simulink model "TLBO_2023"  (R2023b)
settings: Solver=ode45  StartTime=0.0  StopTime=6  MaxStep=1e-4  RelTol=1e-3  EnableMultiTasking=on
PreLoadFcn:
  | Ts_Power=1e-6;
  | Ts_Control=100e-6;
InitFcn:
  | Ts_Power=1e-6;
  | Ts_Control=100e-6;
  | Rtrans=0.142;
  | Xtrans=0.12e-6;
undefined symbols (not defined in the file): DiscIntNeverNeededParam, Ion, Lithium, sigbuilder_block
libraries: dspfdesign x80, spsSeriesRLCBranchLib x52, spsCurrentMeasurementLib x20, spsMeanLib x20, spsIdealSwitchLib x16, spsVoltageMeasurementLib x16, slpidlib x15, spsMosfetLib x14, dspindex x12, spsPWMGeneratorDCDCLib x10, spsGroundLib x10, spsBatteryLib x4
(part 3 of 4)

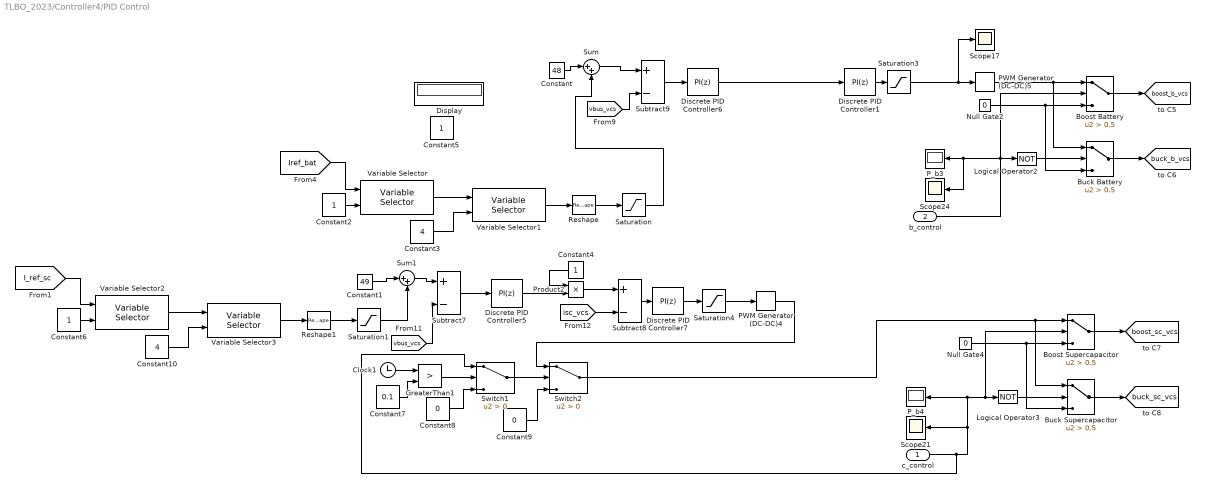
== system TLBO_2023/Controller4/PID Control ==
  c_control : Inport
  b_control : Inport  Port=2
  Boost Battery : Switch  Criteria=u2 > Threshold  Threshold=0.5  SaturateOnIntegerOverflow=off  InputSameDT=off
  Boost Supercapacitor : Switch  Criteria=u2 > Threshold  Threshold=0.5  SaturateOnIntegerOverflow=off  InputSameDT=off
  Buck Battery : Switch  Criteria=u2 > Threshold  Threshold=0.5  SaturateOnIntegerOverflow=off  InputSameDT=off
  Buck Supercapacitor : Switch  Criteria=u2 > Threshold  Threshold=0.5  SaturateOnIntegerOverflow=off  InputSameDT=off
  Clock1 : Clock
  Constant : Constant  Value=48
  Constant1 : Constant  Value=49
  Constant10 : Constant  Value=4
  Constant{2,4..6} (4 alike) : Constant
  Constant3 : Constant  Value=4
  Constant7 : Constant  Value=0.1
  Constant8 : Constant  Value=0
  Constant9 : Constant  Value=0
  Discrete PID Controller1 : slpidlib/PID Controller  Controller=PI  Form=Parallel  TimeDomain=Discrete-time  UseExternalTs=off  SampleTime=-1  IntegratorMethod=Forward Euler  FilterMethod=Forward Euler  ControllerParametersSource=internal  P=0.2  I=4  UseKiTs=off  D=1  N=100  UseFilter=on  TunerSelectOption=Transfer Function Based (PID Tuner App)  InitialConditionSource=internal  InitialConditionForIntegrator=0  InitialConditionForFilter=0  DifferentiatorICPrevScaledInput=0  ExternalReset=none  TrackingMode=off  Kt=1  LimitOutput=off  SatLimitsSource=internal  UpperSaturationLimit=inf  LowerSaturationLimit=-inf  LinearizeAsGain=off  AntiWindupMode=none  Kb=1  LimitIntegrator=off  UpperIntegratorSaturationLimit=inf  LowerIntegratorSaturationLimit=-inf  POutMin=[]  POutMax=[]  IOutMin=[]  IOutMax=[]  DOutMin=[]  DOutMax=[]  NOutMin=[]  NOutMax=[]  SumOutMin=[]  SumOutMax=[]  SaturationOutMin=[]  SaturationOutMax=[]  PParamMin=[]  PParamMax=[]  IParamMin=[]  IParamMax=[]  DParamMin=[]  DParamMax=[]  NParamMin=[]  NParamMax=[]  KbParamMin=[]  KbParamMax=[]  KtParamMin=[]  KtParamMax=[]  KbOutMin=[]  KbOutMax=[]  KtOutMin=[]  KtOutMax=[]  IntegratorOutMin=[]  IntegratorOutMax=[]  FilterOutMin=[]  FilterOutMax=[]  SumI1OutMin=[]  SumI1OutMax=[]  SumI2OutMin=[]  SumI2OutMax=[]  SumI3OutMin=[]  SumI3OutMax=[]  SumI4OutMin=[]  SumI4OutMax=[]  SumDOutMin=[]  SumDOutMax=[]  DifferentiatorOutMin=[]  DifferentiatorOutMax=[]  FilterDiffOutCoefMin=[]  FilterDiffOutCoefMax=[]  ReciprocalOutMin=[]  ReciprocalOutMax=[]  SumDenOutMin=[]  SumDenOutMax=[]  SumNumOutMin=[]  SumNumOutMax=[]  DivideOutMin=[]  DivideOutMax=[]  UdiffTsProdOutMin=[]  UdiffTsProdOutMax=[]  NTsProdOutMin=[]  NTsProdOutMax=[]  UintegralTsProdOutMin=[]  UintegralTsProdOutMax=[]  UngainTsProdOutMin=[]  UngainTsProdOutMax=[]  ClampingZeroOutDataTypeStr=Inherit: Inherit via back propagation  ClampingZeroOutMin=[]  ClampingZeroOutMax=[]  FilterDenConstantOutDataTypeStr=Inherit: Inherit via back propagation  FilterDenConstantOutMin=[]  FilterDenConstantOutMax=[]  PCopyOutDataTypeStr=Inherit: Inherit via back propagation  PCopyOutMin=[]  PCopyOutMax=[]  NCopyOutDataTypeStr=Inherit: Inherit via back propagation  NCopyOutMin=[]  NCopyOutMax=[]  IntegratorContinuousStateAttributes=''  IntegratorStateMustResolveToSignalObject=off  IntegratorRTWStateStorageClass=Auto  FilterContinuousStateAttributes=''  FilterStateMustResolveToSignalObject=off  FilterRTWStateStorageClass=Auto  ParallelPVariant=InternalParameters  IdealPVariant=Disabled  IVariant=InternalParameters  DVariant=Disabled  IntegratorVariant=Discrete  SatVariant=Disabled  AWVariant=Passthrough  PCopyVariant=Disabled  TRVariant=Disabled  FdbkBlocksVariant=Forward  IdealPFdbkVariant=Disabled  SatFdbkVariant=Disabled  DerivativeFilterVariant=Disabled  NVariant=Disabled  NCopyVariant=Disabled_SignalSpec  FilterICVariant=Disabled  IntegratorICVariant=InternalICs  ExternalResetVariant=Disabled  TRSumVariant=Passthrough  SumFdbkVariant=Disabled  SumVariant=Sum_PI  TsampFilterVariant=InternalTs  TsampNgainVariant=Passthrough  TsampIntegralVariant=Disabled_SignalSpec  ExternalSaturationOutDataTypeStr=Inherit: Same as second input
  Discrete PID Controller5 : slpidlib/PID Controller  Controller=PI  Form=Parallel  TimeDomain=Discrete-time  UseExternalTs=off  SampleTime=-1  IntegratorMethod=Forward Euler  FilterMethod=Forward Euler  ControllerParametersSource=internal  P=0  I=4  UseKiTs=off  D=1  N=100  UseFilter=on  TunerSelectOption=Transfer Function Based (PID Tuner App)  InitialConditionSource=internal  InitialConditionForIntegrator=0  InitialConditionForFilter=0  DifferentiatorICPrevScaledInput=0  ExternalReset=none  TrackingMode=off  Kt=1  LimitOutput=off  SatLimitsSource=internal  UpperSaturationLimit=inf  LowerSaturationLimit=-inf  LinearizeAsGain=off  AntiWindupMode=none  Kb=1  LimitIntegrator=off  UpperIntegratorSaturationLimit=inf  LowerIntegratorSaturationLimit=-inf  POutMin=[]  POutMax=[]  IOutMin=[]  IOutMax=[]  DOutMin=[]  DOutMax=[]  NOutMin=[]  NOutMax=[]  SumOutMin=[]  SumOutMax=[]  SaturationOutMin=[]  SaturationOutMax=[]  PParamMin=[]  PParamMax=[]  IParamMin=[]  IParamMax=[]  DParamMin=[]  DParamMax=[]  NParamMin=[]  NParamMax=[]  KbParamMin=[]  KbParamMax=[]  KtParamMin=[]  KtParamMax=[]  KbOutMin=[]  KbOutMax=[]  KtOutMin=[]  KtOutMax=[]  IntegratorOutMin=[]  IntegratorOutMax=[]  FilterOutMin=[]  FilterOutMax=[]  SumI1OutMin=[]  SumI1OutMax=[]  SumI2OutMin=[]  SumI2OutMax=[]  SumI3OutMin=[]  SumI3OutMax=[]  SumI4OutMin=[]  SumI4OutMax=[]  SumDOutMin=[]  SumDOutMax=[]  DifferentiatorOutMin=[]  DifferentiatorOutMax=[]  FilterDiffOutCoefMin=[]  FilterDiffOutCoefMax=[]  ReciprocalOutMin=[]  ReciprocalOutMax=[]  SumDenOutMin=[]  SumDenOutMax=[]  SumNumOutMin=[]  SumNumOutMax=[]  DivideOutMin=[]  DivideOutMax=[]  UdiffTsProdOutMin=[]  UdiffTsProdOutMax=[]  NTsProdOutMin=[]  NTsProdOutMax=[]  UintegralTsProdOutMin=[]  UintegralTsProdOutMax=[]  UngainTsProdOutMin=[]  UngainTsProdOutMax=[]  ClampingZeroOutDataTypeStr=Inherit: Inherit via back propagation  ClampingZeroOutMin=[]  ClampingZeroOutMax=[]  FilterDenConstantOutDataTypeStr=Inherit: Inherit via back propagation  FilterDenConstantOutMin=[]  FilterDenConstantOutMax=[]  PCopyOutDataTypeStr=Inherit: Inherit via back propagation  PCopyOutMin=[]  PCopyOutMax=[]  NCopyOutDataTypeStr=Inherit: Inherit via back propagation  NCopyOutMin=[]  NCopyOutMax=[]  IntegratorContinuousStateAttributes=''  IntegratorStateMustResolveToSignalObject=off  IntegratorRTWStateStorageClass=Auto  FilterContinuousStateAttributes=''  FilterStateMustResolveToSignalObject=off  FilterRTWStateStorageClass=Auto  ParallelPVariant=InternalParameters  IdealPVariant=Disabled  IVariant=InternalParameters  DVariant=Disabled  IntegratorVariant=Discrete  SatVariant=Disabled  AWVariant=Passthrough  PCopyVariant=Disabled  TRVariant=Disabled  FdbkBlocksVariant=Forward  IdealPFdbkVariant=Disabled  SatFdbkVariant=Disabled  DerivativeFilterVariant=Disabled  NVariant=Disabled  NCopyVariant=Disabled_SignalSpec  FilterICVariant=Disabled  IntegratorICVariant=InternalICs  ExternalResetVariant=Disabled  TRSumVariant=Passthrough  SumFdbkVariant=Disabled  SumVariant=Sum_PI  TsampFilterVariant=InternalTs  TsampNgainVariant=Passthrough  TsampIntegralVariant=Disabled_SignalSpec  ExternalSaturationOutDataTypeStr=Inherit: Same as second input
  Discrete PID Controller6 : slpidlib/PID Controller  Controller=PI  Form=Parallel  TimeDomain=Discrete-time  UseExternalTs=off  SampleTime=-1  IntegratorMethod=Forward Euler  FilterMethod=Forward Euler  ControllerParametersSource=internal  P=0  I=1  UseKiTs=off  D=1  N=100  UseFilter=on  TunerSelectOption=Transfer Function Based (PID Tuner App)  InitialConditionSource=internal  InitialConditionForIntegrator=0  InitialConditionForFilter=0  DifferentiatorICPrevScaledInput=0  ExternalReset=none  TrackingMode=off  Kt=1  LimitOutput=off  SatLimitsSource=internal  UpperSaturationLimit=inf  LowerSaturationLimit=-inf  LinearizeAsGain=off  AntiWindupMode=none  Kb=1  LimitIntegrator=off  UpperIntegratorSaturationLimit=inf  LowerIntegratorSaturationLimit=-inf  POutMin=[]  POutMax=[]  IOutMin=[]  IOutMax=[]  DOutMin=[]  DOutMax=[]  NOutMin=[]  NOutMax=[]  SumOutMin=[]  SumOutMax=[]  SaturationOutMin=[]  SaturationOutMax=[]  PParamMin=[]  PParamMax=[]  IParamMin=[]  IParamMax=[]  DParamMin=[]  DParamMax=[]  NParamMin=[]  NParamMax=[]  KbParamMin=[]  KbParamMax=[]  KtParamMin=[]  KtParamMax=[]  KbOutMin=[]  KbOutMax=[]  KtOutMin=[]  KtOutMax=[]  IntegratorOutMin=[]  IntegratorOutMax=[]  FilterOutMin=[]  FilterOutMax=[]  SumI1OutMin=[]  SumI1OutMax=[]  SumI2OutMin=[]  SumI2OutMax=[]  SumI3OutMin=[]  SumI3OutMax=[]  SumI4OutMin=[]  SumI4OutMax=[]  SumDOutMin=[]  SumDOutMax=[]  DifferentiatorOutMin=[]  DifferentiatorOutMax=[]  FilterDiffOutCoefMin=[]  FilterDiffOutCoefMax=[]  ReciprocalOutMin=[]  ReciprocalOutMax=[]  SumDenOutMin=[]  SumDenOutMax=[]  SumNumOutMin=[]  SumNumOutMax=[]  DivideOutMin=[]  DivideOutMax=[]  UdiffTsProdOutMin=[]  UdiffTsProdOutMax=[]  NTsProdOutMin=[]  NTsProdOutMax=[]  UintegralTsProdOutMin=[]  UintegralTsProdOutMax=[]  UngainTsProdOutMin=[]  UngainTsProdOutMax=[]  ClampingZeroOutDataTypeStr=Inherit: Inherit via back propagation  ClampingZeroOutMin=[]  ClampingZeroOutMax=[]  FilterDenConstantOutDataTypeStr=Inherit: Inherit via back propagation  FilterDenConstantOutMin=[]  FilterDenConstantOutMax=[]  PCopyOutDataTypeStr=Inherit: Inherit via back propagation  PCopyOutMin=[]  PCopyOutMax=[]  NCopyOutDataTypeStr=Inherit: Inherit via back propagation  NCopyOutMin=[]  NCopyOutMax=[]  IntegratorContinuousStateAttributes=''  IntegratorStateMustResolveToSignalObject=off  IntegratorRTWStateStorageClass=Auto  FilterContinuousStateAttributes=''  FilterStateMustResolveToSignalObject=off  FilterRTWStateStorageClass=Auto  ParallelPVariant=InternalParameters  IdealPVariant=Disabled  IVariant=InternalParameters  DVariant=Disabled  IntegratorVariant=Discrete  SatVariant=Disabled  AWVariant=Passthrough  PCopyVariant=Disabled  TRVariant=Disabled  FdbkBlocksVariant=Forward  IdealPFdbkVariant=Disabled  SatFdbkVariant=Disabled  DerivativeFilterVariant=Disabled  NVariant=Disabled  NCopyVariant=Disabled_SignalSpec  FilterICVariant=Disabled  IntegratorICVariant=InternalICs  ExternalResetVariant=Disabled  TRSumVariant=Passthrough  SumFdbkVariant=Disabled  SumVariant=Sum_PI  TsampFilterVariant=InternalTs  TsampNgainVariant=Passthrough  TsampIntegralVariant=Disabled_SignalSpec  ExternalSaturationOutDataTypeStr=Inherit: Same as second input
  Discrete PID Controller7 : slpidlib/PID Controller  Controller=PI  Form=Parallel  TimeDomain=Discrete-time  UseExternalTs=off  SampleTime=-1  IntegratorMethod=Forward Euler  FilterMethod=Forward Euler  ControllerParametersSource=internal  P=0.2  I=4  UseKiTs=off  D=1  N=100  UseFilter=on  TunerSelectOption=Transfer Function Based (PID Tuner App)  InitialConditionSource=internal  InitialConditionForIntegrator=0  InitialConditionForFilter=0  DifferentiatorICPrevScaledInput=0  ExternalReset=none  TrackingMode=off  Kt=1  LimitOutput=off  SatLimitsSource=internal  UpperSaturationLimit=inf  LowerSaturationLimit=-inf  LinearizeAsGain=off  AntiWindupMode=none  Kb=1  LimitIntegrator=off  UpperIntegratorSaturationLimit=inf  LowerIntegratorSaturationLimit=-inf  POutMin=[]  POutMax=[]  IOutMin=[]  IOutMax=[]  DOutMin=[]  DOutMax=[]  NOutMin=[]  NOutMax=[]  SumOutMin=[]  SumOutMax=[]  SaturationOutMin=[]  SaturationOutMax=[]  PParamMin=[]  PParamMax=[]  IParamMin=[]  IParamMax=[]  DParamMin=[]  DParamMax=[]  NParamMin=[]  NParamMax=[]  KbParamMin=[]  KbParamMax=[]  KtParamMin=[]  KtParamMax=[]  KbOutMin=[]  KbOutMax=[]  KtOutMin=[]  KtOutMax=[]  IntegratorOutMin=[]  IntegratorOutMax=[]  FilterOutMin=[]  FilterOutMax=[]  SumI1OutMin=[]  SumI1OutMax=[]  SumI2OutMin=[]  SumI2OutMax=[]  SumI3OutMin=[]  SumI3OutMax=[]  SumI4OutMin=[]  SumI4OutMax=[]  SumDOutMin=[]  SumDOutMax=[]  DifferentiatorOutMin=[]  DifferentiatorOutMax=[]  FilterDiffOutCoefMin=[]  FilterDiffOutCoefMax=[]  ReciprocalOutMin=[]  ReciprocalOutMax=[]  SumDenOutMin=[]  SumDenOutMax=[]  SumNumOutMin=[]  SumNumOutMax=[]  DivideOutMin=[]  DivideOutMax=[]  UdiffTsProdOutMin=[]  UdiffTsProdOutMax=[]  NTsProdOutMin=[]  NTsProdOutMax=[]  UintegralTsProdOutMin=[]  UintegralTsProdOutMax=[]  UngainTsProdOutMin=[]  UngainTsProdOutMax=[]  ClampingZeroOutDataTypeStr=Inherit: Inherit via back propagation  ClampingZeroOutMin=[]  ClampingZeroOutMax=[]  FilterDenConstantOutDataTypeStr=Inherit: Inherit via back propagation  FilterDenConstantOutMin=[]  FilterDenConstantOutMax=[]  PCopyOutDataTypeStr=Inherit: Inherit via back propagation  PCopyOutMin=[]  PCopyOutMax=[]  NCopyOutDataTypeStr=Inherit: Inherit via back propagation  NCopyOutMin=[]  NCopyOutMax=[]  IntegratorContinuousStateAttributes=''  IntegratorStateMustResolveToSignalObject=off  IntegratorRTWStateStorageClass=Auto  FilterContinuousStateAttributes=''  FilterStateMustResolveToSignalObject=off  FilterRTWStateStorageClass=Auto  ParallelPVariant=InternalParameters  IdealPVariant=Disabled  IVariant=InternalParameters  DVariant=Disabled  IntegratorVariant=Discrete  SatVariant=Disabled  AWVariant=Passthrough  PCopyVariant=Disabled  TRVariant=Disabled  FdbkBlocksVariant=Forward  IdealPFdbkVariant=Disabled  SatFdbkVariant=Disabled  DerivativeFilterVariant=Disabled  NVariant=Disabled  NCopyVariant=Disabled_SignalSpec  FilterICVariant=Disabled  IntegratorICVariant=InternalICs  ExternalResetVariant=Disabled  TRSumVariant=Passthrough  SumFdbkVariant=Disabled  SumVariant=Sum_PI  TsampFilterVariant=InternalTs  TsampNgainVariant=Passthrough  TsampIntegralVariant=Disabled_SignalSpec  ExternalSaturationOutDataTypeStr=Inherit: Same as second input
  Display : Display
  GreaterThan1 : RelationalOperator  Operator=>  OutDataTypeStr=boolean  RndMeth=Simplest  InputSameDT=off
  Logical Operator2 : Logic  Operator=NOT  AllPortsSameDT=off  OutDataTypeStr=boolean
  Logical Operator3 : Logic  Operator=NOT  AllPortsSameDT=off  OutDataTypeStr=boolean
  Null Gate2 : Constant  Value=0
  Null Gate4 : Constant  Value=0
  PWM Generator (DC-DC)4 : spsPWMGeneratorDCDCLib/PWM Generator (DC-DC)  Fsw=10e3  Ts=0
  PWM Generator (DC-DC)5 : spsPWMGeneratorDCDCLib/PWM Generator (DC-DC)  Fsw=10e3  Ts=0
  P_b3 : Display
      settings: Format=binary (Stored Integer)  Decimation=1000
  P_b4 : Display
      settings: Format=binary (Stored Integer)  Decimation=1000
  Product2 : Product
  Reshape : Reshape
  Reshape1 : Reshape
  Saturation : Saturate
  Saturation1 : Saturate
  Saturation3 : Saturate  UpperLimit=0.8  LowerLimit=0  ZeroCross=off
  Saturation4 : Saturate  UpperLimit=0.8  LowerLimit=0  ZeroCross=off
  Scope17 : Scope
  Scope21 : Scope
  Scope24 : Scope
  Subtract7 : Sum  Inputs=+-
  Subtract8 : Sum  Inputs=+-
  Subtract9 : Sum  Inputs=+-
  Sum : Sum  Inputs=|++
  Sum1 : Sum  Inputs=|++
  Switch1 : Switch  Criteria=u2 > Threshold  SaturateOnIntegerOverflow=off  InputSameDT=off
  Switch2 : Switch  Criteria=u2 > Threshold  SaturateOnIntegerOverflow=off  InputSameDT=off
  Variable Selector : dspindex/Variable Selector  NumInputs=1  rowsOrCols=Rows  IdxMode=Variable  Elements=[1 3]  ZerOneIdxMode=One-based  errmode=Clip Index  FillMode=on  FillValues=0
  Variable Selector1 : dspindex/Variable Selector  NumInputs=1  rowsOrCols=Columns  IdxMode=Variable  Elements=[1 3]  ZerOneIdxMode=One-based  errmode=Clip Index  FillMode=on  FillValues=0
  Variable Selector2 : dspindex/Variable Selector  NumInputs=1  rowsOrCols=Rows  IdxMode=Variable  Elements=[1 3]  ZerOneIdxMode=One-based  errmode=Clip Index  FillMode=on  FillValues=0
  Variable Selector3 : dspindex/Variable Selector  NumInputs=1  rowsOrCols=Columns  IdxMode=Variable  Elements=[1 3]  ZerOneIdxMode=One-based  errmode=Clip Index  FillMode=on  FillValues=0
  tag scope: boost_b_vcs=global, boost_sc_vcs=global, buck_b_vcs=global, buck_sc_vcs=global
  wires:
  Buck Battery/1 -> [buck_b_vcs]
  Null Gate2/1 -> Boost Battery/3, Buck Battery/3
  b_control/1 -> Scope24/1, P_b3/1, Logical Operator2/1, Boost Battery/2
  Boost Battery/1 -> [boost_b_vcs]
  PWM Generator (DC-DC)5/1 -> Buck Battery/1, Boost Battery/1
  Logical Operator2/1 -> Buck Battery/2
  [vbus_vcs] -> Subtract9/2
  Buck Supercapacitor/1 -> [buck_sc_vcs]
  Null Gate4/1 -> Buck Supercapacitor/3, Boost Supercapacitor/3
  Boost Supercapacitor/1 -> [boost_sc_vcs]
  Subtract7/1 -> Discrete PID Controller5/1
  [vbus_vcs] -> Subtract7/2
  Saturation4/1 -> PWM Generator (DC-DC)4/1
  Saturation3/1 -> Scope17/1, PWM Generator (DC-DC)5/1
  [isc_vcs] -> Subtract8/2
  Product2/1 -> Subtract8/1
  Discrete PID Controller5/1 -> Product2/2
  Constant4/1 -> Product2/1
  Subtract8/1 -> Discrete PID Controller7/1
  Discrete PID Controller7/1 -> Saturation4/1
  Subtract9/1 -> Discrete PID Controller6/1
  Discrete PID Controller1/1 -> Saturation3/1
  Reshape/1 -> Saturation/1
  Variable Selector/1 -> Variable Selector1/1
  Constant3/1 -> Variable Selector1/2
  [Iref_bat] -> Variable Selector/1
  Variable Selector1/1 -> Reshape/1
  Constant2/1 -> Variable Selector/2
  Discrete PID Controller6/1 -> Discrete PID Controller1/1
  Constant/1 -> Sum/1
  Sum/1 -> Subtract9/1
  c_control/1 -> Switch1/1, Scope21/1, P_b4/1, Boost Supercapacitor/2, Logical Operator3/1
  Logical Operator3/1 -> Buck Supercapacitor/2
  PWM Generator (DC-DC)4/1 -> Switch2/1
  GreaterThan1/1 -> Switch1/2
  Clock1/1 -> GreaterThan1/1
  Constant9/1 -> Switch2/3
  Constant8/1 -> Switch1/3
  Constant7/1 -> GreaterThan1/2
  Switch1/1 -> Switch2/2
  Switch2/1 -> Buck Supercapacitor/1, Boost Supercapacitor/1
  Saturation/1 -> Sum/2
  Variable Selector3/1 -> Reshape1/1
  Reshape1/1 -> Saturation1/1
  Variable Selector2/1 -> Variable Selector3/1
  Constant10/1 -> Variable Selector3/2
  Constant6/1 -> Variable Selector2/2
  [I_ref_sc] -> Variable Selector2/1
  Constant1/1 -> Sum1/1
  Saturation1/1 -> Sum1/2
  Sum1/1 -> Subtract7/1

== system TLBO_2023/DC Load 1_2/Load Control ==
  Demux : Demux  Tag=STV Demux  Outputs=5
      settings: DisplayOption=none
  FromWs : FromWorkspace  Tag=STV FromWs  VariableName=tuvar
      SigBuilderData=|
      | common.afterFinalStr = 'Extrapolate'
      | common.sampleTime = '0'
      | dataSet(1).timeRange = [0 6]
      | dataSet(1).name = 'Constant Irradiance'
      | dataSet(2).timeRange = [0 6]
      | dataSet(2).name = 'Step Irradiance'
      | dataSet(3).timeRange = [0 6]
      | dataSet(3).name = 'Load Switch Control'
      | sbobj.Groups(1).Name = 'Constant Irradiance'
      | sbobj.Groups(1).Signals(1).Name = 'S1'
      | sbobj.Groups(1).Signals(1).XData = [0 6]
      | sbobj.Groups(1).Signals(1).YData = [1000 1000]
      | sbobj.Groups(1).Signals(2).Name = 'S2'
      | sbobj.Groups(1).Signals(2).XData = [0 3 3 6]
      | sbobj.Groups(1).Signals(2).YData = [0 0 1 1]
      | sbobj.Groups(1).Signals(3).Name = 'S3'
      | sbobj.Groups(1).Signals(3).XData = [0 3 3 6]
      | sbobj.Groups(1).Signals(3).YData = [0 0 1 1]
      | sbobj.Groups(1).Signals(4).Name = 'S4'
      | sbobj.Groups(1).Signals(4).XData = [0 3 3 6]
      | sbobj.Groups(1).Signals(4).YData = [0 0 1 1]
      | sbobj.Groups(1).Signals(5).Name = 'Signal 1'
      | sbobj.Groups(1).Signals(5).XData = [0 6]
      | sbobj.Groups(1).Signals(5).YData = [0 0]
      | sbobj.Groups(1).TimeRange = [0 6]
      | sbobj.Groups(2).Name = 'Step Irradiance'
      | sbobj.Groups(2).Signals(1).Name = 'S1'
      | sbobj.Groups(2).Signals(1).XData = [0 0.252 0.252 6]
      | sbobj.Groups(2).Signals(1).YData = [600 600 1000 1000]
      | sbobj.Groups(2).Signals(2).Name = 'S2'
      | sbobj.Groups(2).Signals(2).XData = [0 3 3 6]
      | sbobj.Groups(2).Signals(2).YData = [0 0 1 1]
      | sbobj.Groups(2).Signals(3).Name = 'S3'
      | sbobj.Groups(2).Signals(3).XData = [0 3 3 6]
      | sbobj.Groups(2).Signals(3).YData = [0 0 1 1]
      | sbobj.Groups(2).Signals(4).Name = 'S4'
      | sbobj.Groups(2).Signals(4).XData = [0 3 3 6]
      | sbobj.Groups(2).Signals(4).YData = [0 0 1 1]
      | sbobj.Groups(2).Signals(5).Name = 'Signal 1'
      | sbobj.Groups(2).Signals(5).XData = [0 6]
      | sbobj.Groups(2).Signals(5).YData = [0 0]
      | sbobj.Groups(2).TimeRange = [0 6]
      | sbobj.Groups(3).Name = 'Load Switch Control'
      | sbobj.Groups(3).Signals(1).Name = 'S1'
      | sbobj.Groups(3).Signals(1).XData = [0 2.995 2.995 3.995 3.995 6]
      | sbobj.Groups(3).Signals(1).YData = [-0.01 -0.01 1 1 0 0]
      | sbobj.Groups(3).Signals(2).Name = 'S2'
      | sbobj.Groups(3).Signals(2).XData = [0 2 3 6]
      | sbobj.Groups(3).Signals(2).YData = [0 0 0 0]
      | sbobj.Groups(3).Signals(3).Name = 'S3'
      | sbobj.Groups(3).Signals(3).XData = [0 3 3 4 4 6]
      | sbobj.Groups(3).Signals(3).YData = [0 0 1 1 0 0]
      | sbobj.Groups(3).Signals(4).Name = 'S4'
      | sbobj.Groups(3).Signals(4).XData = [0 3 4 5 6]
      | sbobj.Groups(3).Signals(4).YData = [0 0 0 0 0]
      | sbobj.Groups(3).Signals(5).Name = 'Signal 1'
      | sbobj.Groups(3).Signals(5).XData = [0 6]
      | sbobj.Groups(3).Signals(5).YData = [0 0]
      | sbobj.Groups(3).TimeRange = [0 6]
  S1 : Outport  Tag=STV Outport  VectorParamsAs1DForOutWhenUnconnected=off
  S2 : Outport  Tag=STV Outport  Port=2  VectorParamsAs1DForOutWhenUnconnected=off
  S3 : Outport  Tag=STV Outport  Port=3  VectorParamsAs1DForOutWhenUnconnected=off
  S4 : Outport  Tag=STV Outport  Port=4  VectorParamsAs1DForOutWhenUnconnected=off
  Signal 1 : Outport  Tag=STV Outport  Port=5
  wires:
  Demux/1 -> S1/1
  FromWs/1 -> Demux/1
  Demux/2 -> S2/1
  Demux/3 -> S3/1
  Demux/4 -> S4/1
  Demux/5 -> Signal 1/1

== system TLBO_2023/DC Load 1_4/Load Control ==
  Demux : Demux  Tag=STV Demux  Outputs=5
      settings: DisplayOption=none
  FromWs : FromWorkspace  Tag=STV FromWs  VariableName=tuvar
      SigBuilderData=|
      | common.afterFinalStr = 'Extrapolate'
      | common.sampleTime = '0'
      | dataSet(1).timeRange = [0 6]
      | dataSet(1).name = 'Constant Irradiance'
      | dataSet(2).timeRange = [0 6]
      | dataSet(2).name = 'Step Irradiance'
      | dataSet(3).timeRange = [0 6]
      | dataSet(3).name = 'Load Switch Control'
      | sbobj.Groups(1).Name = 'Constant Irradiance'
      | sbobj.Groups(1).Signals(1).Name = 'S1'
      | sbobj.Groups(1).Signals(1).XData = [0 6]
      | sbobj.Groups(1).Signals(1).YData = [1000 1000]
      | sbobj.Groups(1).Signals(2).Name = 'S2'
      | sbobj.Groups(1).Signals(2).XData = [0 3 3 6]
      | sbobj.Groups(1).Signals(2).YData = [0 0 1 1]
      | sbobj.Groups(1).Signals(3).Name = 'S3'
      | sbobj.Groups(1).Signals(3).XData = [0 3 3 6]
      | sbobj.Groups(1).Signals(3).YData = [0 0 1 1]
      | sbobj.Groups(1).Signals(4).Name = 'S4'
      | sbobj.Groups(1).Signals(4).XData = [0 3 3 6]
      | sbobj.Groups(1).Signals(4).YData = [0 0 1 1]
      | sbobj.Groups(1).Signals(5).Name = 'Signal 1'
      | sbobj.Groups(1).Signals(5).XData = [0 6]
      | sbobj.Groups(1).Signals(5).YData = [0 0]
      | sbobj.Groups(1).TimeRange = [0 6]
      | sbobj.Groups(2).Name = 'Step Irradiance'
      | sbobj.Groups(2).Signals(1).Name = 'S1'
      | sbobj.Groups(2).Signals(1).XData = [0 0.252 0.252 6]
      | sbobj.Groups(2).Signals(1).YData = [600 600 1000 1000]
      | sbobj.Groups(2).Signals(2).Name = 'S2'
      | sbobj.Groups(2).Signals(2).XData = [0 3 3 6]
      | sbobj.Groups(2).Signals(2).YData = [0 0 1 1]
      | sbobj.Groups(2).Signals(3).Name = 'S3'
      | sbobj.Groups(2).Signals(3).XData = [0 3 3 6]
      | sbobj.Groups(2).Signals(3).YData = [0 0 1 1]
      | sbobj.Groups(2).Signals(4).Name = 'S4'
      | sbobj.Groups(2).Signals(4).XData = [0 3 3 6]
      | sbobj.Groups(2).Signals(4).YData = [0 0 1 1]
      | sbobj.Groups(2).Signals(5).Name = 'Signal 1'
      | sbobj.Groups(2).Signals(5).XData = [0 6]
      | sbobj.Groups(2).Signals(5).YData = [0 0]
      | sbobj.Groups(2).TimeRange = [0 6]
      | sbobj.Groups(3).Name = 'Load Switch Control'
      | sbobj.Groups(3).Signals(1).Name = 'S1'
      | sbobj.Groups(3).Signals(1).XData = [0 0.06 0.06 0.99 0.99 6]
      | sbobj.Groups(3).Signals(1).YData = [-0.01 -0.01 0.99 1.01 0 0]
      | sbobj.Groups(3).Signals(2).Name = 'S2'
      | sbobj.Groups(3).Signals(2).XData = [0 2 3 6]
      | sbobj.Groups(3).Signals(2).YData = [0 0 0 0]
      | sbobj.Groups(3).Signals(3).Name = 'S3'
      | sbobj.Groups(3).Signals(3).XData = [0 3 3 4 4 6]
      | sbobj.Groups(3).Signals(3).YData = [0 0 1 1 0 0]
      | sbobj.Groups(3).Signals(4).Name = 'S4'
      | sbobj.Groups(3).Signals(4).XData = [0 3 4 5 6]
      | sbobj.Groups(3).Signals(4).YData = [0 0 0 0 0]
      | sbobj.Groups(3).Signals(5).Name = 'Signal 1'
      | sbobj.Groups(3).Signals(5).XData = [0 6]
      | sbobj.Groups(3).Signals(5).YData = [0 0]
      | sbobj.Groups(3).TimeRange = [0 6]
  S1 : Outport  Tag=STV Outport  VectorParamsAs1DForOutWhenUnconnected=off
  S2 : Outport  Tag=STV Outport  Port=2  VectorParamsAs1DForOutWhenUnconnected=off
  S3 : Outport  Tag=STV Outport  Port=3  VectorParamsAs1DForOutWhenUnconnected=off
  S4 : Outport  Tag=STV Outport  Port=4  VectorParamsAs1DForOutWhenUnconnected=off
  Signal 1 : Outport  Tag=STV Outport  Port=5
  wires:
  Demux/1 -> S1/1
  FromWs/1 -> Demux/1
  Demux/2 -> S2/1
  Demux/3 -> S3/1
  Demux/4 -> S4/1
  Demux/5 -> Signal 1/1

== system TLBO_2023/DC Load 2_3/Load Control ==
  Demux : Demux  Tag=STV Demux  Outputs=5
      settings: DisplayOption=none
  FromWs : FromWorkspace  Tag=STV FromWs  VariableName=tuvar
      SigBuilderData=|
      | common.afterFinalStr = 'Extrapolate'
      | common.sampleTime = '0'
      | dataSet(1).timeRange = [0 6]
      | dataSet(1).name = 'Constant Irradiance'
      | dataSet(2).timeRange = [0 6]
      | dataSet(2).name = 'Step Irradiance'
      | dataSet(3).timeRange = [0 6]
      | dataSet(3).name = 'Load Switch Control'
      | sbobj.Groups(1).Name = 'Constant Irradiance'
      | sbobj.Groups(1).Signals(1).Name = 'S1'
      | sbobj.Groups(1).Signals(1).XData = [0 6]
      | sbobj.Groups(1).Signals(1).YData = [1000 1000]
      | sbobj.Groups(1).Signals(2).Name = 'S2'
      | sbobj.Groups(1).Signals(2).XData = [0 3 3 6]
      | sbobj.Groups(1).Signals(2).YData = [0 0 1 1]
      | sbobj.Groups(1).Signals(3).Name = 'S3'
      | sbobj.Groups(1).Signals(3).XData = [0 3 3 6]
      | sbobj.Groups(1).Signals(3).YData = [0 0 1 1]
      | sbobj.Groups(1).Signals(4).Name = 'S4'
      | sbobj.Groups(1).Signals(4).XData = [0 3 3 6]
      | sbobj.Groups(1).Signals(4).YData = [0 0 1 1]
      | sbobj.Groups(1).Signals(5).Name = 'Signal 1'
      | sbobj.Groups(1).Signals(5).XData = [0 6]
      | sbobj.Groups(1).Signals(5).YData = [0 0]
      | sbobj.Groups(1).TimeRange = [0 6]
      | sbobj.Groups(2).Name = 'Step Irradiance'
      | sbobj.Groups(2).Signals(1).Name = 'S1'
      | sbobj.Groups(2).Signals(1).XData = [0 0.252 0.252 6]
      | sbobj.Groups(2).Signals(1).YData = [600 600 1000 1000]
      | sbobj.Groups(2).Signals(2).Name = 'S2'
      | sbobj.Groups(2).Signals(2).XData = [0 3 3 6]
      | sbobj.Groups(2).Signals(2).YData = [0 0 1 1]
      | sbobj.Groups(2).Signals(3).Name = 'S3'
      | sbobj.Groups(2).Signals(3).XData = [0 3 3 6]
      | sbobj.Groups(2).Signals(3).YData = [0 0 1 1]
      | sbobj.Groups(2).Signals(4).Name = 'S4'
      | sbobj.Groups(2).Signals(4).XData = [0 3 3 6]
      | sbobj.Groups(2).Signals(4).YData = [0 0 1 1]
      | sbobj.Groups(2).Signals(5).Name = 'Signal 1'
      | sbobj.Groups(2).Signals(5).XData = [0 6]
      | sbobj.Groups(2).Signals(5).YData = [0 0]
      | sbobj.Groups(2).TimeRange = [0 6]
      | sbobj.Groups(3).Name = 'Load Switch Control'
      | sbobj.Groups(3).Signals(1).Name = 'S1'
      | sbobj.Groups(3).Signals(1).XData = [0 2.005 2.005 3.01 3.01 6]
      | sbobj.Groups(3).Signals(1).YData = [-0.01 -0.01 1 1.01 0 0]
      | sbobj.Groups(3).Signals(2).Name = 'S2'
      | sbobj.Groups(3).Signals(2).XData = [0 2 3 6]
      | sbobj.Groups(3).Signals(2).YData = [0 0 0 0]
      | sbobj.Groups(3).Signals(3).Name = 'S3'
      | sbobj.Groups(3).Signals(3).XData = [0 3 3 4 4 6]
      | sbobj.Groups(3).Signals(3).YData = [0 0 1 1 0 0]
      | sbobj.Groups(3).Signals(4).Name = 'S4'
      | sbobj.Groups(3).Signals(4).XData = [0 3 4 5 6]
      | sbobj.Groups(3).Signals(4).YData = [0 0 0 0 0]
      | sbobj.Groups(3).Signals(5).Name = 'Signal 1'
      | sbobj.Groups(3).Signals(5).XData = [0 6]
      | sbobj.Groups(3).Signals(5).YData = [0 0]
      | sbobj.Groups(3).TimeRange = [0 6]
  S1 : Outport  Tag=STV Outport  VectorParamsAs1DForOutWhenUnconnected=off
  S2 : Outport  Tag=STV Outport  Port=2  VectorParamsAs1DForOutWhenUnconnected=off
  S3 : Outport  Tag=STV Outport  Port=3  VectorParamsAs1DForOutWhenUnconnected=off
  S4 : Outport  Tag=STV Outport  Port=4  VectorParamsAs1DForOutWhenUnconnected=off
  Signal 1 : Outport  Tag=STV Outport  Port=5
  wires:
  Demux/1 -> S1/1
  FromWs/1 -> Demux/1
  Demux/2 -> S2/1
  Demux/3 -> S3/1
  Demux/4 -> S4/1
  Demux/5 -> Signal 1/1

== system TLBO_2023/DC Load 3_4/Load Control ==
  Demux : Demux  Tag=STV Demux  Outputs=5
      settings: DisplayOption=none
  FromWs : FromWorkspace  Tag=STV FromWs  VariableName=tuvar
      SigBuilderData=|
      | common.afterFinalStr = 'Extrapolate'
      | common.sampleTime = '0'
      | dataSet(1).timeRange = [0 6]
      | dataSet(1).name = 'Constant Irradiance'
      | dataSet(2).timeRange = [0 6]
      | dataSet(2).name = 'Step Irradiance'
      | dataSet(3).timeRange = [0 6]
      | dataSet(3).name = 'Load Switch Control'
      | sbobj.Groups(1).Name = 'Constant Irradiance'
      | sbobj.Groups(1).Signals(1).Name = 'S1'
      | sbobj.Groups(1).Signals(1).XData = [0 6]
      | sbobj.Groups(1).Signals(1).YData = [1000 1000]
      | sbobj.Groups(1).Signals(2).Name = 'S2'
      | sbobj.Groups(1).Signals(2).XData = [0 3 3 6]
      | sbobj.Groups(1).Signals(2).YData = [0 0 1 1]
      | sbobj.Groups(1).Signals(3).Name = 'S3'
      | sbobj.Groups(1).Signals(3).XData = [0 3 3 6]
      | sbobj.Groups(1).Signals(3).YData = [0 0 1 1]
      | sbobj.Groups(1).Signals(4).Name = 'S4'
      | sbobj.Groups(1).Signals(4).XData = [0 3 3 6]
      | sbobj.Groups(1).Signals(4).YData = [0 0 1 1]
      | sbobj.Groups(1).Signals(5).Name = 'Signal 1'
      | sbobj.Groups(1).Signals(5).XData = [0 6]
      | sbobj.Groups(1).Signals(5).YData = [0 0]
      | sbobj.Groups(1).TimeRange = [0 6]
      | sbobj.Groups(2).Name = 'Step Irradiance'
      | sbobj.Groups(2).Signals(1).Name = 'S1'
      | sbobj.Groups(2).Signals(1).XData = [0 0.252 0.252 6]
      | sbobj.Groups(2).Signals(1).YData = [600 600 1000 1000]
      | sbobj.Groups(2).Signals(2).Name = 'S2'
      | sbobj.Groups(2).Signals(2).XData = [0 3 3 6]
      | sbobj.Groups(2).Signals(2).YData = [0 0 1 1]
      | sbobj.Groups(2).Signals(3).Name = 'S3'
      | sbobj.Groups(2).Signals(3).XData = [0 3 3 6]
      | sbobj.Groups(2).Signals(3).YData = [0 0 1 1]
      | sbobj.Groups(2).Signals(4).Name = 'S4'
      | sbobj.Groups(2).Signals(4).XData = [0 3 3 6]
      | sbobj.Groups(2).Signals(4).YData = [0 0 1 1]
      | sbobj.Groups(2).Signals(5).Name = 'Signal 1'
      | sbobj.Groups(2).Signals(5).XData = [0 6]
      | sbobj.Groups(2).Signals(5).YData = [0 0]
      | sbobj.Groups(2).TimeRange = [0 6]
      | sbobj.Groups(3).Name = 'Load Switch Control'
      | sbobj.Groups(3).Signals(1).Name = 'S1'
      | sbobj.Groups(3).Signals(1).XData = [0 1 1 1.995 1.995 6]
      | sbobj.Groups(3).Signals(1).YData = [-0.01 -0.01 0.99 1.01 0 0]
      | sbobj.Groups(3).Signals(2).Name = 'S2'
      | sbobj.Groups(3).Signals(2).XData = [0 2 3 6]
      | sbobj.Groups(3).Signals(2).YData = [0 0 0 0]
      | sbobj.Groups(3).Signals(3).Name = 'S3'
      | sbobj.Groups(3).Signals(3).XData = [0 3 3 4 4 6]
      | sbobj.Groups(3).Signals(3).YData = [0 0 1 1 0 0]
      | sbobj.Groups(3).Signals(4).Name = 'S4'
      | sbobj.Groups(3).Signals(4).XData = [0 3 4 5 6]
      | sbobj.Groups(3).Signals(4).YData = [0 0 0 0 0]
      | sbobj.Groups(3).Signals(5).Name = 'Signal 1'
      | sbobj.Groups(3).Signals(5).XData = [0 6]
      | sbobj.Groups(3).Signals(5).YData = [0 0]
      | sbobj.Groups(3).TimeRange = [0 6]
  S1 : Outport  Tag=STV Outport  VectorParamsAs1DForOutWhenUnconnected=off
  S2 : Outport  Tag=STV Outport  Port=2  VectorParamsAs1DForOutWhenUnconnected=off
  S3 : Outport  Tag=STV Outport  Port=3  VectorParamsAs1DForOutWhenUnconnected=off
  S4 : Outport  Tag=STV Outport  Port=4  VectorParamsAs1DForOutWhenUnconnected=off
  Signal 1 : Outport  Tag=STV Outport  Port=5
  wires:
  Demux/1 -> S1/1
  FromWs/1 -> Demux/1
  Demux/2 -> S2/1
  Demux/3 -> S3/1
  Demux/4 -> S4/1
  Demux/5 -> Signal 1/1

== system TLBO_2023/Source1/Battery Storage ==
  {1..5} (5 alike) : dspfdesign/Analog Filter Design  method=Butterworth  filttype=Lowpass  N=8  Wlo=pi*50  Whi=80  Rp=2  Rs=40
  Battery : spsBatteryLib/Battery  BatType=Lithium-Ion  NomV=12  NomQ=42  SOC=50  Batt_Tr=30  PresetModel=on  MaxQ=42  MinV=9  FullV=13.9678  Dis_rate=18.2609  R=0.0028571  Normal_OP=37.9826  expZone="[12.9646      2.06348]"
  Bus Selector1 : BusSelector  OutputSignals=SOC (%),Current (A),Voltage (V)
  Current Measurement : spsCurrentMeasurementLib/Current Measurement  PhasorSimulation=off  OutputType=Complex  PSBequivalent=0
  Ground1 : spsGroundLib/Ground  LConnTagsString=a
  Mosfet : spsMosfetLib/Mosfet  Ron=0.1  Lon=0  Rd=0.01  Vfd=0  IC=0  Rs=1e5  Cs=inf  Measurements=on
  Mosfet1 : spsMosfetLib/Mosfet  Ron=0.1  Lon=0  Rd=0.01  Vfd=0  IC=0  Rs=1e5  Cs=inf  Measurements=on
  Product1 : Product
  Scope1 : Scope  NumInputPorts=2
  Scope2 : Scope  NumInputPorts=2
  Series RLC Branch : spsSeriesRLCBranchLib/Series RLC Branch  LConnTagsString=__new0  RConnTagsString=__new0  BranchType=RL  Resistance=0.02  Inductance=150e-6  SetiL0=off  InitialCurrent=0  Capacitance=1e-6  Setx0=off  InitialVoltage=0  Measurements=None
  Series RLC Branch1 : spsSeriesRLCBranchLib/Series RLC Branch  LConnTagsString=__new0  RConnTagsString=__new0  BranchType=RC  Resistance=0.02  Inductance=1e-3  SetiL0=off  InitialCurrent=0  Capacitance=220e-6  Setx0=off  InitialVoltage=0  Measurements=None
  Voltage Measurement2 : spsVoltageMeasurementLib/Voltage Measurement  PhasorSimulation=off  OutputType=Complex  PSBequivalent=0
  + : PMIOPort  Side=Right
  - : PMIOPort  Port=2  Side=Right
  SOC : Outport  VectorParamsAs1DForOutWhenUnconnected=off
  Power : Outport  Port=2  VectorParamsAs1DForOutWhenUnconnected=off
  tag scope: ib_pv=global, soc_b_pv=global, vb_pv=global
  wires:
  Current Measurement/1 -> 4/1
  3/1 -> Scope1/1
  1/1 -> Scope1/2
  Battery/1 -> Bus Selector1/1
  2/1 -> Scope2/2
  4/1 -> Scope2/1
  Voltage Measurement2/1 -> 2/1
  [buck_b_pv] -> Mosfet1/1
  [boost_b_pv] -> Mosfet/1
  Bus Selector1/2 -> [ib_pv], 3/1, Product1/1  "<Current (A)>"
  Bus Selector1/1 -> [soc_b_pv], SOC/1  "<SOC (%)>"
  Bus Selector1/3 -> Product1/2, [vb_pv], 1/1  "<Voltage (V)>"
  5/1 -> Power/1
  Product1/1 -> 5/1
  connections:
  Battery/LConn1 -- Series RLC Branch/LConn1
  Mosfet/RConn1 -- Ground1/LConn1 -- Series RLC Branch1/RConn1 -- Voltage Measurement2/LConn2 -- -/RConn1 -- Battery/LConn2
  Mosfet/LConn1 -- Mosfet1/RConn1 -- Series RLC Branch/RConn1
  Mosfet1/LConn1 -- Voltage Measurement2/LConn1 -- Current Measurement/LConn1 -- Series RLC Branch1/LConn1
  +/RConn1 -- Current Measurement/RConn1

== system TLBO_2023/Source1/Rooftop Solar System ==
  2 : dspfdesign/Analog Filter Design  method=Butterworth  filttype=Lowpass  N=8  Wlo=pi*50  Whi=80  Rp=2  Rs=40
  C3 : spsSeriesRLCBranchLib/Series RLC Branch  LConnTagsString=__new0  RConnTagsString=__new0  BranchType=C  Resistance=1.0  Inductance=1.0  SetiL0=off  InitialCurrent=0  Capacitance=100e-6  Setx0=off  InitialVoltage=0  Measurements=Branch voltage
  Current Measurement : spsCurrentMeasurementLib/Current Measurement  PhasorSimulation=off  OutputType=Complex  PSBequivalent=0
  Diode1 : spsDiodeLib/Diode  Ron=1e-4  Lon=0  Vf=0  IC=0  UseSnubber=off  Rs=inf  Cs=inf  Measurements=off
  Irradiance (W/m^2) : Display
      settings: Format=bank  Decimation=1000
  Irradiance Temp : Subsystem  Tag=STV Subsys  LoadFcn=sigbuilder_block('load');  StartFcn=sigbuilder_block('start');  StopFcn=sigbuilder_block('stop');  ClipboardFcn=sigbuilder_block('clipboard');  mask(Sigbuilder block){tuvar=[0:10]}
      mask help: Sigbuilder GUI
      mask init:
      | if ~strcmp(get_param(bdroot(gcbh),'SimulationStatus'),'stopped') tuvar = sigbuilder_block('maskInit'); end
      settings: CopyFcn=sigbuilder_block('copy');  DeleteFcn=sigbuilder_block('delete');  ModelCloseFcn=sigbuilder_block('modelClose');  PreSaveFcn=sigbuilder_block('preSave');  PauseFcn=sigbuilder_block('pause')  ContinueFcn=sigbuilder_block('continue')  NameChangeFcn=sigbuilder_block('namechange');  OpenFcn=sigbuilder_block('open',[0 0 1152 591.6 ]);  CloseFcn=sigbuilder_block('close');
      mask Display: plot(0, 0, 100, 100,[2, 2, 32, 32, 2], [68, 8, 8, 68, 68],[32, 2], [38, 38], [32, 19, 2],[53, 60, 44], [32, 17, 17, 2],[16, 16, 31, 31]);txt = getActiveGroup(gcbh);text(2, 100, txt,'verticalAlignment', 'top');
  L1 : spsSeriesRLCBranchLib/Series RLC Branch  LConnTagsString=__new0  RConnTagsString=__new0  BranchType=RL  Resistance=0.005  Inductance=150e-6  SetiL0=off  InitialCurrent=0  Capacitance=1e-6  Setx0=off  InitialVoltage=0  Measurements=None
  MPPT : Subsystem  mask(Boost Control - MPPT){fc=10e3, T_MPPT=200e-6, Dinit=0.5}
      mask prompts: fc "PWM switching frequency (Hz)"; T_MPPT "Time window used by MPPT control (s)"; Dinit "Initial value of duty cycle"
  Mosfet : spsMosfetLib/Mosfet  Ron=0.1  Lon=0  Rd=0.01  Vfd=0  IC=0  Rs=1e5  Cs=inf  Measurements=on
  "P (kW) " : Display
      settings: Format=bank  Decimation=2000
  PV : Scope  NumInputPorts=5
  Pmean : Subsystem
  Product : Product
  Rooftop-Solar Solar : spsPVArrayLib/PV Array  Npar=4  Nser=2  PlotType=array @ 25 deg.C & specified irradiances  S_vec="[ 1000  500  250 ]"  Temp_C_vec=[ 25 ]  ModuleName=User-defined  PlotWhenSelected=off  Pm=243.412  Ncell=60  Voc=38.3  Isc=8.81  Vm=30.2  Im=8.06  beta_Voc_pc=-0.35601  alpha_Isc_pc=0.07  beta_Voc=-0.13635  alpha_Isc=0.006167  IL=8.8468  I0=2.613e-10  nI=1.0265  Rsh=103.8804  Rs=0.43387  RobustModel=off  RobustCellTemperature=25  BAL=on  Tc=1e-6  Tfilter=5e-5
      settings: AttributesFormatString=|
      | %<ModuleName>
      | %<Nser>-module string
      | %<Npar> parallel strings
  Scope1 : Scope  NumInputPorts=3
  Scope3 : Scope  NumInputPorts=2
  Subsystem1 : Subsystem
      mask Display: disp('Open this block\nto display additional \nscopes & measurements')
  Temperature (deg. C) : Display
      settings: Format=bank  Decimation=1000
  Vdc 1 : spsVoltageMeasurementLib/Voltage Measurement  Tag=PoWeRsYsTeMmEaSuReMeNt  PhasorSimulation=off  OutputType=Magnitude  PSBequivalent=0
  Vdc Boost : Display
      settings: Format=bank  Decimation=2000
  powergui : spspowerguiLib/powergui  Priority=1  SimulationMode=Continuous  SampleTime=Ts_Power  frequency=60  Iterations=50  frequencyindice=0  Pbase=100e6  ErrMax=1e-4  UnitsV=kV  UnitsW=MW  buscounter=0  FunctionMessages=off  echomessages=off  EnableUseOfTLC=off  CurrentSourceSwitches=off  DisableSnubberDevices=off  DisableRonSwitches=off  DisableVfSwitches=off  DisplayEquations=off  AutomaticDiscreteSolvers=off  SolverType=Tustin/Backward Euler (TBE)  Interpol=off  ExternalGateDelay=off  methode=off  Ts=100  x0status=blocks  SPID=on  SwTol=0  HookPort=off  NonlinearTolerance=1e-4  nMaxIteration=100  ContinueOnMaxIteration=off  RestoreLinks=warning  ResistiveCurrentMeasurement=off  Frange=[0:2:500]  Ylog=off  Xlog=on  ShowGrid=off  save=off  variable=ZData  structure=0  ZoomFFT=on  StartTime=0.0  cycles=1  DisplayStyle=1  fundamental=60  FreqAxis=off  MaxFrequency=1000  frequencyindicesteady=1  RmsSteady=1  display=off
  + : PMIOPort  Side=Right
  - : PMIOPort  Port=2  Side=Right
  Power : Outport  VectorParamsAs1DForOutWhenUnconnected=off
  tag scope: m_PV=global
  wires:
  2/1 -> Power/1, Scope1/3
  Pmean/1(P) -> PV/3, "P (kW) "/1  "Pmean  (kW)"
  Pmean/2(V) -> PV/4, Vdc Boost/1  "Vmean (V)"
  Rooftop-Solar Solar/1 -> [m_PV]
  [D] -> PV/5  "Duty Cycle"
  [Temp] -> PV/2  "Temp (deg. C)"
  [Ir] -> PV/1  "Ir (W/m^2)"
  Vdc 1/1 -> Product/2, Scope1/2
  Current Measurement/1 -> Product/1, Scope1/1
  [V_PV] -> Scope3/1, MPPT/1(V_PV)
  [I_PV] -> Scope3/2, MPPT/2(I_PV)
  Irradiance Temp/1(Ir) -> Rooftop-Solar Solar/1, Irradiance (W/m^2)/1
  Irradiance Temp/2(Temp) -> Rooftop-Solar Solar/2, Temperature (deg. C)/1
  MPPT/1(Pulses) -> Mosfet/1
  Product/1 -> 2/1
  connections:
  Mosfet/LConn1 -- L1/RConn1 -- Diode1/LConn1
  Rooftop-Solar Solar/RConn2 -- Vdc 1/LConn2 -- C3/RConn1 -- -/RConn1 -- Mosfet/RConn1
  L1/LConn1 -- C3/LConn1 -- Current Measurement/RConn1
  Vdc 1/LConn1 -- Rooftop-Solar Solar/RConn1 -- Current Measurement/LConn1
  +/RConn1 -- Diode1/RConn1

== system TLBO_2023/Source2/Battery Storage ==
  {1..5} (5 alike) : dspfdesign/Analog Filter Design  method=Butterworth  filttype=Lowpass  N=8  Wlo=pi*50  Whi=80  Rp=2  Rs=40
  Battery : spsBatteryLib/Battery  BatType=Lithium-Ion  NomV=12  NomQ=42  SOC=50  Batt_Tr=30  PresetModel=on  MaxQ=42  MinV=9  FullV=13.9678  Dis_rate=18.2609  R=0.0028571  Normal_OP=37.9826  expZone="[12.9646      2.06348]"
  Bus Selector1 : BusSelector  OutputSignals=SOC (%),Current (A),Voltage (V)
  Current Measurement : spsCurrentMeasurementLib/Current Measurement  PhasorSimulation=off  OutputType=Complex  PSBequivalent=0
  Ground1 : spsGroundLib/Ground  LConnTagsString=a
  Mosfet : spsMosfetLib/Mosfet  Ron=0.1  Lon=0  Rd=0.01  Vfd=0  IC=0  Rs=1e5  Cs=inf  Measurements=on
  Mosfet1 : spsMosfetLib/Mosfet  Ron=0.1  Lon=0  Rd=0.01  Vfd=0  IC=0  Rs=1e5  Cs=inf  Measurements=on
  Product1 : Product
  Scope1 : Scope  NumInputPorts=2
  Scope2 : Scope  NumInputPorts=2
  Series RLC Branch : spsSeriesRLCBranchLib/Series RLC Branch  LConnTagsString=__new0  RConnTagsString=__new0  BranchType=RL  Resistance=0.02  Inductance=150e-6  SetiL0=off  InitialCurrent=0  Capacitance=1e-6  Setx0=off  InitialVoltage=0  Measurements=None
  Series RLC Branch1 : spsSeriesRLCBranchLib/Series RLC Branch  LConnTagsString=__new0  RConnTagsString=__new0  BranchType=RC  Resistance=0.02  Inductance=1e-3  SetiL0=off  InitialCurrent=0  Capacitance=220e-6  Setx0=off  InitialVoltage=0  Measurements=None
  Voltage Measurement2 : spsVoltageMeasurementLib/Voltage Measurement  PhasorSimulation=off  OutputType=Complex  PSBequivalent=0
  + : PMIOPort  Side=Right
  - : PMIOPort  Port=2  Side=Right
  SOC : Outport  VectorParamsAs1DForOutWhenUnconnected=off
  Power : Outport  Port=2  VectorParamsAs1DForOutWhenUnconnected=off
  tag scope: ib_pv2=global, soc_b_pv2=global, vb_pv2=global
  wires:
  Current Measurement/1 -> 4/1
  3/1 -> Scope1/1
  1/1 -> Scope1/2
  Battery/1 -> Bus Selector1/1
  2/1 -> Scope2/2
  4/1 -> Scope2/1
  Voltage Measurement2/1 -> 2/1
  [buck_b_pv2] -> Mosfet1/1
  [boost_b_pv2] -> Mosfet/1
  Bus Selector1/2 -> [ib_pv2], 3/1, Product1/1  "<Current (A)>"
  Bus Selector1/1 -> [soc_b_pv2], SOC/1  "<SOC (%)>"
  Bus Selector1/3 -> Product1/2, [vb_pv2], 1/1  "<Voltage (V)>"
  5/1 -> Power/1
  Product1/1 -> 5/1
  connections:
  Battery/LConn1 -- Series RLC Branch/LConn1
  Mosfet/RConn1 -- Ground1/LConn1 -- Series RLC Branch1/RConn1 -- Voltage Measurement2/LConn2 -- -/RConn1 -- Battery/LConn2
  Mosfet/LConn1 -- Mosfet1/RConn1 -- Series RLC Branch/RConn1
  Mosfet1/LConn1 -- Voltage Measurement2/LConn1 -- Current Measurement/LConn1 -- Series RLC Branch1/LConn1
  +/RConn1 -- Current Measurement/RConn1

== system TLBO_2023/Source2/Rooftop Solar System ==
  2 : dspfdesign/Analog Filter Design  method=Butterworth  filttype=Lowpass  N=8  Wlo=pi*50  Whi=80  Rp=2  Rs=40
  C3 : spsSeriesRLCBranchLib/Series RLC Branch  LConnTagsString=__new0  RConnTagsString=__new0  BranchType=C  Resistance=1.0  Inductance=1.0  SetiL0=off  InitialCurrent=0  Capacitance=100e-6  Setx0=off  InitialVoltage=0  Measurements=Branch voltage
  Current Measurement : spsCurrentMeasurementLib/Current Measurement  PhasorSimulation=off  OutputType=Complex  PSBequivalent=0
  Diode1 : spsDiodeLib/Diode  Ron=1e-4  Lon=0  Vf=0  IC=0  UseSnubber=off  Rs=inf  Cs=inf  Measurements=off
  Irradiance (W/m^2) : Display
      settings: Format=bank  Decimation=1000
  Irradiance Temp : Subsystem  Tag=STV Subsys  LoadFcn=sigbuilder_block('load');  StartFcn=sigbuilder_block('start');  StopFcn=sigbuilder_block('stop');  ClipboardFcn=sigbuilder_block('clipboard');  mask(Sigbuilder block){tuvar=[0:10]}
      mask help: Sigbuilder GUI
      mask init:
      | if ~strcmp(get_param(bdroot(gcbh),'SimulationStatus'),'stopped') tuvar = sigbuilder_block('maskInit'); end
      settings: CopyFcn=sigbuilder_block('copy');  DeleteFcn=sigbuilder_block('delete');  ModelCloseFcn=sigbuilder_block('modelClose');  PreSaveFcn=sigbuilder_block('preSave');  PauseFcn=sigbuilder_block('pause')  ContinueFcn=sigbuilder_block('continue')  NameChangeFcn=sigbuilder_block('namechange');  OpenFcn=sigbuilder_block('open',[0 0 1152 591.6 ]);  CloseFcn=sigbuilder_block('close');
      mask Display: plot(0, 0, 100, 100,[2, 2, 32, 32, 2], [68, 8, 8, 68, 68],[32, 2], [38, 38], [32, 19, 2],[53, 60, 44], [32, 17, 17, 2],[16, 16, 31, 31]);txt = getActiveGroup(gcbh);text(2, 100, txt,'verticalAlignment', 'top');
  L1 : spsSeriesRLCBranchLib/Series RLC Branch  LConnTagsString=__new0  RConnTagsString=__new0  BranchType=RL  Resistance=0.005  Inductance=150e-6  SetiL0=off  InitialCurrent=0  Capacitance=1e-6  Setx0=off  InitialVoltage=0  Measurements=None
  MPPT : Subsystem  mask(Boost Control - MPPT){fc=10e3, T_MPPT=200e-6, Dinit=0.5}
      mask prompts: fc "PWM switching frequency (Hz)"; T_MPPT "Time window used by MPPT control (s)"; Dinit "Initial value of duty cycle"
  Mosfet : spsMosfetLib/Mosfet  Ron=0.1  Lon=0  Rd=0.01  Vfd=0  IC=0  Rs=1e5  Cs=inf  Measurements=on
  "P (kW) " : Display
      settings: Format=bank  Decimation=2000
  PV : Scope  NumInputPorts=5
  Pmean : Subsystem
  Product : Product
  Rooftop-Solar Solar : spsPVArrayLib/PV Array  Npar=4  Nser=2  PlotType=array @ 25 deg.C & specified irradiances  S_vec="[ 1000  500  250 ]"  Temp_C_vec=[ 25 ]  ModuleName=User-defined  PlotWhenSelected=off  Pm=243.412  Ncell=60  Voc=38.3  Isc=8.81  Vm=30.2  Im=8.06  beta_Voc_pc=-0.35601  alpha_Isc_pc=0.07  beta_Voc=-0.13635  alpha_Isc=0.006167  IL=8.8468  I0=2.613e-10  nI=1.0265  Rsh=103.8804  Rs=0.43387  RobustModel=off  RobustCellTemperature=25  BAL=on  Tc=1e-6  Tfilter=5e-5
      settings: AttributesFormatString=|
      | %<ModuleName>
      | %<Nser>-module string
      | %<Npar> parallel strings
  Scope1 : Scope  NumInputPorts=3
  Scope3 : Scope  NumInputPorts=2
  Subsystem1 : Subsystem
      mask Display: disp('Open this block\nto display additional \nscopes & measurements')
  Temperature (deg. C) : Display
      settings: Format=bank  Decimation=1000
  Vdc 1 : spsVoltageMeasurementLib/Voltage Measurement  Tag=PoWeRsYsTeMmEaSuReMeNt  PhasorSimulation=off  OutputType=Magnitude  PSBequivalent=0
  Vdc Boost : Display
      settings: Format=bank  Decimation=2000
  powergui : spspowerguiLib/powergui  Priority=1  SimulationMode=Continuous  SampleTime=Ts_Power  frequency=60  Iterations=50  frequencyindice=0  Pbase=100e6  ErrMax=1e-4  UnitsV=kV  UnitsW=MW  buscounter=0  FunctionMessages=off  echomessages=off  EnableUseOfTLC=off  CurrentSourceSwitches=off  DisableSnubberDevices=off  DisableRonSwitches=off  DisableVfSwitches=off  DisplayEquations=off  AutomaticDiscreteSolvers=off  SolverType=Tustin/Backward Euler (TBE)  Interpol=off  ExternalGateDelay=off  methode=off  Ts=100  x0status=blocks  SPID=on  SwTol=0  HookPort=off  NonlinearTolerance=1e-4  nMaxIteration=100  ContinueOnMaxIteration=off  RestoreLinks=warning  ResistiveCurrentMeasurement=off  Frange=[0:2:500]  Ylog=off  Xlog=on  ShowGrid=off  save=off  variable=ZData  structure=0  ZoomFFT=on  StartTime=0.0  cycles=1  DisplayStyle=1  fundamental=60  FreqAxis=off  MaxFrequency=1000  frequencyindicesteady=1  RmsSteady=1  display=off
  + : PMIOPort  Side=Right
  - : PMIOPort  Port=2  Side=Right
  Power : Outport  VectorParamsAs1DForOutWhenUnconnected=off
  tag scope: m_PV2=global
  wires:
  2/1 -> Power/1, Scope1/3
  Pmean/1(P) -> PV/3, "P (kW) "/1  "Pmean  (kW)"
  Pmean/2(V) -> PV/4, Vdc Boost/1  "Vmean (V)"
  Rooftop-Solar Solar/1 -> [m_PV2]
  [D2] -> PV/5  "Duty Cycle"
  [Temp2] -> PV/2  "Temp (deg. C)"
  [Ir2] -> PV/1  "Ir (W/m^2)"
  Vdc 1/1 -> Product/2, Scope1/2
  Current Measurement/1 -> Product/1, Scope1/1
  [V_PV2] -> Scope3/1, MPPT/1(V_PV2)
  [I_PV2] -> Scope3/2, MPPT/2(I_PV2)
  Irradiance Temp/1(Ir) -> Rooftop-Solar Solar/1, Irradiance (W/m^2)/1
  Irradiance Temp/2(Temp) -> Rooftop-Solar Solar/2, Temperature (deg. C)/1
  MPPT/1(Pulses) -> Mosfet/1
  Product/1 -> 2/1
  connections:
  Mosfet/LConn1 -- L1/RConn1 -- Diode1/LConn1
  Rooftop-Solar Solar/RConn2 -- Vdc 1/LConn2 -- C3/RConn1 -- -/RConn1 -- Mosfet/RConn1
  L1/LConn1 -- C3/LConn1 -- Current Measurement/RConn1
  Vdc 1/LConn1 -- Rooftop-Solar Solar/RConn1 -- Current Measurement/LConn1
  +/RConn1 -- Diode1/RConn1

== system TLBO_2023/Source3/Battery Storage ==
  {1..5} (5 alike) : dspfdesign/Analog Filter Design  method=Butterworth  filttype=Lowpass  N=8  Wlo=pi*50  Whi=80  Rp=2  Rs=40
  Battery : spsBatteryLib/Battery  BatType=Lithium-Ion  NomV=24  NomQ=42  SOC=50  Batt_Tr=30  PresetModel=on  MaxQ=42  MinV=18  FullV=27.9357  Dis_rate=18.2609  R=0.0057143  Normal_OP=37.9826  expZone="[25.9293      2.06348]"
  Bus Selector1 : BusSelector  OutputSignals=SOC (%),Current (A),Voltage (V)
  Current Measurement : spsCurrentMeasurementLib/Current Measurement  PhasorSimulation=off  OutputType=Complex  PSBequivalent=0
  Ground1 : spsGroundLib/Ground  LConnTagsString=a
  Mosfet : spsMosfetLib/Mosfet  Ron=0.1  Lon=0  Rd=0.01  Vfd=0  IC=0  Rs=1e5  Cs=inf  Measurements=on
  Mosfet1 : spsMosfetLib/Mosfet  Ron=0.1  Lon=0  Rd=0.01  Vfd=0  IC=0  Rs=1e5  Cs=inf  Measurements=on
  Product1 : Product
  Scope1 : Scope  NumInputPorts=2
  Scope2 : Scope  NumInputPorts=2
  Series RLC Branch : spsSeriesRLCBranchLib/Series RLC Branch  LConnTagsString=__new0  RConnTagsString=__new0  BranchType=RL  Resistance=0.02  Inductance=150e-6  SetiL0=off  InitialCurrent=0  Capacitance=1e-6  Setx0=off  InitialVoltage=0  Measurements=None
  Series RLC Branch1 : spsSeriesRLCBranchLib/Series RLC Branch  LConnTagsString=__new0  RConnTagsString=__new0  BranchType=RC  Resistance=0.02  Inductance=1e-3  SetiL0=off  InitialCurrent=0  Capacitance=220e-6  Setx0=off  InitialVoltage=0  Measurements=None
  Voltage Measurement2 : spsVoltageMeasurementLib/Voltage Measurement  PhasorSimulation=off  OutputType=Complex  PSBequivalent=0
  + : PMIOPort  Side=Right
  - : PMIOPort  Port=2  Side=Right
  SOC : Outport  VectorParamsAs1DForOutWhenUnconnected=off
  Power : Outport  Port=2  VectorParamsAs1DForOutWhenUnconnected=off
  tag scope: ib_pcs=global, soc_b_pcs=global, vb_pcs=global
  wires:
  Product1/1 -> 5/1
  5/1 -> Power/1
  Bus Selector1/3 -> 1/1, [vb_pcs], Product1/2  "<Voltage (V)>"
  Bus Selector1/1 -> SOC/1, [soc_b_pcs]  "<SOC (%)>"
  Bus Selector1/2 -> Product1/1, 3/1, [ib_pcs]  "<Current (A)>"
  [boost_b_pcs] -> Mosfet/1
  [buck_b_pcs] -> Mosfet1/1
  Voltage Measurement2/1 -> 2/1
  4/1 -> Scope2/1
  2/1 -> Scope2/2
  Battery/1 -> Bus Selector1/1
  1/1 -> Scope1/2
  3/1 -> Scope1/1
  Current Measurement/1 -> 4/1
  connections:
  +/RConn1 -- Current Measurement/RConn1
  Series RLC Branch1/LConn1 -- Current Measurement/LConn1 -- Voltage Measurement2/LConn1 -- Mosfet1/LConn1
  Series RLC Branch/RConn1 -- Mosfet1/RConn1 -- Mosfet/LConn1
  Battery/LConn2 -- -/RConn1 -- Voltage Measurement2/LConn2 -- Series RLC Branch1/RConn1 -- Ground1/LConn1 -- Mosfet/RConn1
  Battery/LConn1 -- Series RLC Branch/LConn1

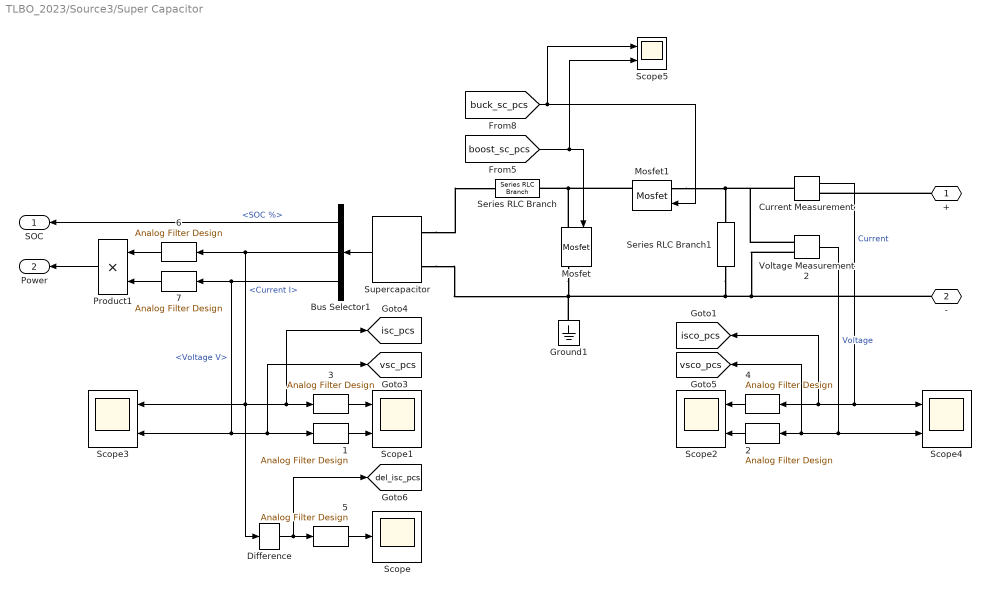
== system TLBO_2023/Source3/Super Capacitor ==
  {1..7} (7 alike) : dspfdesign/Analog Filter Design  method=Butterworth  filttype=Lowpass  N=8  Wlo=pi*50  Whi=80  Rp=2  Rs=40
  Bus Selector1 : BusSelector  OutputSignals=SOC %,Current I,Voltage V
  Current Measurement : spsCurrentMeasurementLib/Current Measurement  PhasorSimulation=off  OutputType=Complex  PSBequivalent=0
  Difference : simulink/Discrete/Difference  ICPrevInput=0.0  OutMin=[]  OutMax=[]  OutDataType=fixdt(1, 16)  OutScaling=2^-10  DoSatur=off
  Ground1 : spsGroundLib/Ground  LConnTagsString=a
  Mosfet : spsMosfetLib/Mosfet  Ron=0.1  Lon=0  Rd=0.01  Vfd=0  IC=0  Rs=1e5  Cs=inf  Measurements=on
  Mosfet1 : spsMosfetLib/Mosfet  Ron=0.1  Lon=0  Rd=0.01  Vfd=0  IC=0  Rs=1e5  Cs=inf  Measurements=on
  Product1 : Product
  Scope : Scope
  Scope{1..5} (5 alike) : Scope  NumInputPorts=2
  Series RLC Branch : spsSeriesRLCBranchLib/Series RLC Branch  LConnTagsString=__new0  RConnTagsString=__new0  BranchType=RL  Resistance=0.02  Inductance=150e-6  SetiL0=off  InitialCurrent=0  Capacitance=1e-6  Setx0=off  InitialVoltage=0  Measurements=None
  Series RLC Branch1 : spsSeriesRLCBranchLib/Series RLC Branch  LConnTagsString=__new0  RConnTagsString=__new0  BranchType=RC  Resistance=0.02  Inductance=1e-3  SetiL0=off  InitialCurrent=0  Capacitance=220e-6  Setx0=off  InitialVoltage=0  Measurements=None
  Supercapacitor : spsSupercapacitorLib/Supercapacitor  C=58  Rdc=8.9e-3  Voltage=16  Ns=1  Np=1  Vinit=16  Temp=25  Nc=1  r=1e-9  epsilon=6.0208e-10  Ioc=10  Vself="[48  47.8  47.06  44.65]"
  Voltage Measurement2 : spsVoltageMeasurementLib/Voltage Measurement  PhasorSimulation=off  OutputType=Complex  PSBequivalent=0
  + : PMIOPort  Side=Right
  - : PMIOPort  Port=2  Side=Right
  SOC : Outport  VectorParamsAs1DForOutWhenUnconnected=off
  Power : Outport  Port=2  VectorParamsAs1DForOutWhenUnconnected=off
  tag scope: del_isc_pcs=global, isc_pcs=global, isco_pcs=global, vsc_pcs=global, vsco_pcs=global
  wires:
  3/1 -> Scope1/1
  1/1 -> Scope1/2
  Supercapacitor/1 -> Bus Selector1/1
  2/1 -> Scope2/2
  4/1 -> Scope2/1
  Voltage Measurement2/1 -> [vsco_pcs], 2/1, Scope4/2  "Voltage"
  [buck_sc_pcs] -> Scope5/1, Mosfet1/1
  [boost_sc_pcs] -> Scope5/2, Mosfet/1
  Current Measurement/1 -> [isco_pcs], 4/1, Scope4/1  "Current"
  Difference/1 -> 5/1, [del_isc_pcs]
  5/1 -> Scope/1
  Product1/1 -> Power/1
  Bus Selector1/2 -> 6/1, Difference/1, [isc_pcs], 3/1, Scope3/1  "<Current I>"
  Bus Selector1/1 -> SOC/1  "<SOC %>"
  Bus Selector1/3 -> 7/1, Scope3/2, [vsc_pcs], 1/1  "<Voltage V>"
  6/1 -> Product1/1
  7/1 -> Product1/2
  connections:
  Supercapacitor/LConn1 -- Series RLC Branch/LConn1
  Voltage Measurement2/LConn2 -- Series RLC Branch1/RConn1 -- Supercapacitor/LConn2 -- Mosfet/RConn1 -- Ground1/LConn1 -- -/RConn1
  Mosfet/LConn1 -- Mosfet1/RConn1 -- Series RLC Branch/RConn1
  Mosfet1/LConn1 -- Voltage Measurement2/LConn1 -- Current Measurement/LConn1 -- Series RLC Branch1/LConn1
  +/RConn1 -- Current Measurement/RConn1

== system TLBO_2023/Source4/Battery Storage ==
  {1..5} (5 alike) : dspfdesign/Analog Filter Design  method=Butterworth  filttype=Lowpass  N=8  Wlo=pi*50  Whi=80  Rp=2  Rs=40
  Battery : spsBatteryLib/Battery  BatType=Lithium-Ion  NomV=12  NomQ=42  SOC=50  Batt_Tr=30  PresetModel=on  MaxQ=42  MinV=9  FullV=13.9678  Dis_rate=18.2609  R=0.0028571  Normal_OP=37.9826  expZone="[12.9646      2.06348]"
  Bus Selector1 : BusSelector  OutputSignals=SOC (%),Current (A),Voltage (V)
  Current Measurement : spsCurrentMeasurementLib/Current Measurement  PhasorSimulation=off  OutputType=Complex  PSBequivalent=0
  DC Voltage Source : spsDCVoltageSourceLib/DC Voltage Source  Amplitude=0  Measurements=None
  Ground1 : spsGroundLib/Ground  LConnTagsString=a
  Mosfet : spsMosfetLib/Mosfet  Ron=0.1  Lon=0  Rd=0.01  Vfd=0  IC=0  Rs=1e5  Cs=inf  Measurements=on
  Mosfet1 : spsMosfetLib/Mosfet  Ron=0.1  Lon=0  Rd=0.01  Vfd=0  IC=0  Rs=1e5  Cs=inf  Measurements=on
  Product1 : Product
  Scope1 : Scope  NumInputPorts=2
  Scope2 : Scope  NumInputPorts=2
  Series RLC Branch : spsSeriesRLCBranchLib/Series RLC Branch  LConnTagsString=__new0  RConnTagsString=__new0  BranchType=RL  Resistance=0.02  Inductance=150e-6  SetiL0=off  InitialCurrent=0  Capacitance=1e-6  Setx0=off  InitialVoltage=0  Measurements=None
  Series RLC Branch1 : spsSeriesRLCBranchLib/Series RLC Branch  LConnTagsString=__new0  RConnTagsString=__new0  BranchType=RC  Resistance=0.02  Inductance=1e-3  SetiL0=off  InitialCurrent=0  Capacitance=220e-6  Setx0=off  InitialVoltage=0  Measurements=None
  Voltage Measurement2 : spsVoltageMeasurementLib/Voltage Measurement  PhasorSimulation=off  OutputType=Complex  PSBequivalent=0
  + : PMIOPort  Side=Right
  - : PMIOPort  Port=2  Side=Right
  SOC : Outport  VectorParamsAs1DForOutWhenUnconnected=off
  Power : Outport  Port=2  VectorParamsAs1DForOutWhenUnconnected=off
  tag scope: ib_vcs=global, soc_b_vcs=global, vb_vcs=global
  wires:
  Current Measurement/1 -> 4/1
  3/1 -> Scope1/1
  1/1 -> Scope1/2
  Battery/1 -> Bus Selector1/1
  2/1 -> Scope2/2
  4/1 -> Scope2/1
  Voltage Measurement2/1 -> 2/1
  [buck_b_vcs] -> Mosfet1/1
  [boost_b_vcs] -> Mosfet/1
  Bus Selector1/2 -> [ib_vcs], 3/1, Product1/1  "<Current (A)>"
  Bus Selector1/1 -> [soc_b_vcs], SOC/1  "<SOC (%)>"
  Bus Selector1/3 -> Product1/2, [vb_vcs], 1/1  "<Voltage (V)>"
  5/1 -> Power/1
  Product1/1 -> 5/1
  connections:
  DC Voltage Source/RConn1 -- Series RLC Branch/LConn1
  Mosfet/RConn1 -- Ground1/LConn1 -- Series RLC Branch1/RConn1 -- Voltage Measurement2/LConn2 -- -/RConn1 -- Battery/LConn2
  Mosfet/LConn1 -- Mosfet1/RConn1 -- Series RLC Branch/RConn1
  Mosfet1/LConn1 -- Voltage Measurement2/LConn1 -- Current Measurement/LConn1 -- Series RLC Branch1/LConn1
  +/RConn1 -- Current Measurement/RConn1
  DC Voltage Source/LConn1 -- Battery/LConn1

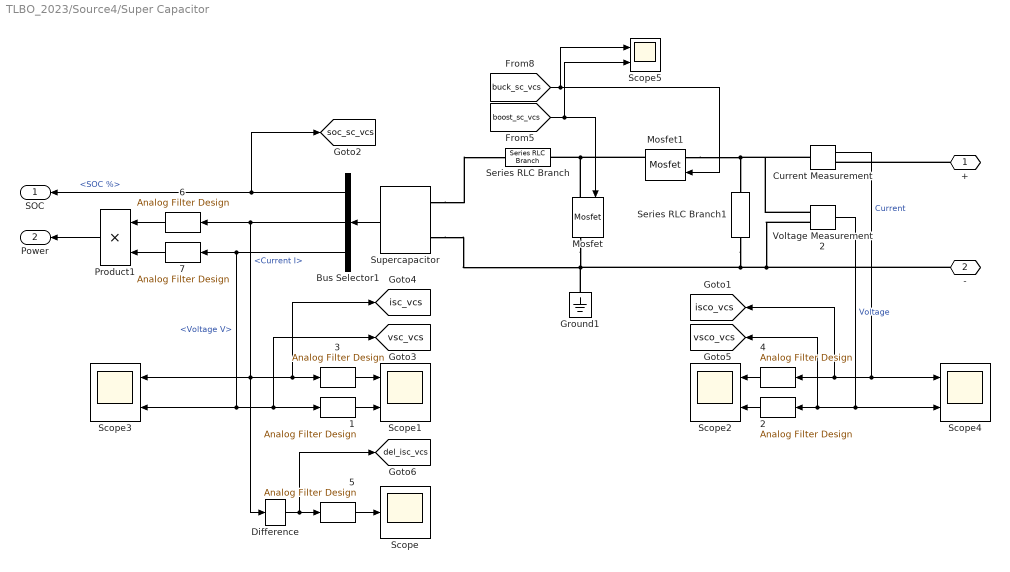
== system TLBO_2023/Source4/Super Capacitor ==
  {1..7} (7 alike) : dspfdesign/Analog Filter Design  method=Butterworth  filttype=Lowpass  N=8  Wlo=pi*50  Whi=80  Rp=2  Rs=40
  Bus Selector1 : BusSelector  OutputSignals=SOC %,Current I,Voltage V
  Current Measurement : spsCurrentMeasurementLib/Current Measurement  PhasorSimulation=off  OutputType=Complex  PSBequivalent=0
  Difference : simulink/Discrete/Difference  ICPrevInput=0.0  OutMin=[]  OutMax=[]  OutDataType=fixdt(1, 16)  OutScaling=2^-10  DoSatur=off
  Ground1 : spsGroundLib/Ground  LConnTagsString=a
  Mosfet : spsMosfetLib/Mosfet  Ron=0.1  Lon=0  Rd=0.01  Vfd=0  IC=0  Rs=1e5  Cs=inf  Measurements=on
  Mosfet1 : spsMosfetLib/Mosfet  Ron=0.1  Lon=0  Rd=0.01  Vfd=0  IC=0  Rs=1e5  Cs=inf  Measurements=on
  Product1 : Product
  Scope : Scope
  Scope{1..5} (5 alike) : Scope  NumInputPorts=2
  Series RLC Branch : spsSeriesRLCBranchLib/Series RLC Branch  LConnTagsString=__new0  RConnTagsString=__new0  BranchType=RL  Resistance=0.02  Inductance=150e-6  SetiL0=off  InitialCurrent=0  Capacitance=1e-6  Setx0=off  InitialVoltage=0  Measurements=None
  Series RLC Branch1 : spsSeriesRLCBranchLib/Series RLC Branch  LConnTagsString=__new0  RConnTagsString=__new0  BranchType=RC  Resistance=0.02  Inductance=1e-3  SetiL0=off  InitialCurrent=0  Capacitance=220e-6  Setx0=off  InitialVoltage=0  Measurements=None
  Supercapacitor : spsSupercapacitorLib/Supercapacitor  C=58  Rdc=8.9e-3  Voltage=16  Ns=1  Np=1  Vinit=16  Temp=25  Nc=1  r=1e-9  epsilon=6.0208e-10  Ioc=10  Vself="[48  47.8  47.06  44.65]"
  Voltage Measurement2 : spsVoltageMeasurementLib/Voltage Measurement  PhasorSimulation=off  OutputType=Complex  PSBequivalent=0
  + : PMIOPort  Side=Right
  - : PMIOPort  Port=2  Side=Right
  SOC : Outport  VectorParamsAs1DForOutWhenUnconnected=off
  Power : Outport  Port=2  VectorParamsAs1DForOutWhenUnconnected=off
  tag scope: del_isc_vcs=global, isc_vcs=global, isco_vcs=global, soc_sc_vcs=global, vsc_vcs=global, vsco_vcs=global
  wires:
  3/1 -> Scope1/1
  1/1 -> Scope1/2
  Supercapacitor/1 -> Bus Selector1/1
  2/1 -> Scope2/2
  4/1 -> Scope2/1
  Voltage Measurement2/1 -> [vsco_vcs], 2/1, Scope4/2  "Voltage"
  [buck_sc_vcs] -> Scope5/1, Mosfet1/1
  [boost_sc_vcs] -> Scope5/2, Mosfet/1
  Current Measurement/1 -> [isco_vcs], 4/1, Scope4/1  "Current"
  Difference/1 -> 5/1, [del_isc_vcs]
  5/1 -> Scope/1
  Product1/1 -> Power/1
  Bus Selector1/2 -> 6/1, Difference/1, [isc_vcs], 3/1, Scope3/1  "<Current I>"
  Bus Selector1/1 -> SOC/1, [soc_sc_vcs]  "<SOC %>"
  Bus Selector1/3 -> 7/1, Scope3/2, [vsc_vcs], 1/1  "<Voltage V>"
  6/1 -> Product1/1
  7/1 -> Product1/2
  connections:
  Supercapacitor/LConn1 -- Series RLC Branch/LConn1
  Voltage Measurement2/LConn2 -- Series RLC Branch1/RConn1 -- Supercapacitor/LConn2 -- Mosfet/RConn1 -- Ground1/LConn1 -- -/RConn1
  Mosfet/LConn1 -- Mosfet1/RConn1 -- Series RLC Branch/RConn1
  Mosfet1/LConn1 -- Voltage Measurement2/LConn1 -- Current Measurement/LConn1 -- Series RLC Branch1/LConn1
  +/RConn1 -- Current Measurement/RConn1

== system TLBO_2023/Source1/Rooftop Solar System/Irradiance Temp ==
  Demux : Demux  Tag=STV Demux  Outputs=2
      settings: DisplayOption=none
  FromWs : FromWorkspace  Tag=STV FromWs  VariableName=tuvar
      SigBuilderData=|
      | common.afterFinalStr = 'Extrapolate'
      | common.sampleTime = '0'
      | dataSet(1).timeRange = [0 2]
      | dataSet(1).name = 'Constant Irradiance'
      | dataSet(2).timeRange = [0 2]
      | dataSet(2).name = 'Step Irradiance'
      | dataSet(3).timeRange = [0 6]
      | dataSet(3).name = 'Ramp-up/down Irradiance'
      | sbobj.Groups(1).Name = 'Constant Irradiance'
      | sbobj.Groups(1).Signals(1).Name = 'Ir'
      | sbobj.Groups(1).Signals(1).XData = [0 2]
      | sbobj.Groups(1).Signals(1).YData = [1000 1000]
      | sbobj.Groups(1).Signals(2).Name = 'Temp'
      | sbobj.Groups(1).Signals(2).XData = [0 1 1 2]
      | sbobj.Groups(1).Signals(2).YData = [0 0 1 1]
      | sbobj.Groups(1).TimeRange = [0 2]
      | sbobj.Groups(2).Name = 'Step Irradiance'
      | sbobj.Groups(2).Signals(1).Name = 'Ir'
      | sbobj.Groups(2).Signals(1).XData = [0 0.252 0.252 2]
      | sbobj.Groups(2).Signals(1).YData = [600 600 1000 1000]
      | sbobj.Groups(2).Signals(2).Name = 'Temp'
      | sbobj.Groups(2).Signals(2).XData = [0 1 1 2]
      | sbobj.Groups(2).Signals(2).YData = [0 0 1 1]
      | sbobj.Groups(2).TimeRange = [0 2]
      | sbobj.Groups(3).Name = 'Ramp-up/down Irradiance'
      | sbobj.Groups(3).Signals(1).Name = 'Ir'
      | sbobj.Groups(3).Signals(1).XData = [0 0.6 1.1 2.2 2.7 6]
      | sbobj.Groups(3).Signals(1).YData = [1000 1000 250 250 1000 1000]
      | sbobj.Groups(3).Signals(2).Name = 'Temp'
      | sbobj.Groups(3).Signals(2).XData = [0 1.5 2.2 3 3.7 6]
      | sbobj.Groups(3).Signals(2).YData = [25 25 28 28 25 25]
      | sbobj.Groups(3).TimeRange = [0 6]
  Ir : Outport  Tag=STV Outport  VectorParamsAs1DForOutWhenUnconnected=off
  Temp : Outport  Tag=STV Outport  Port=2  VectorParamsAs1DForOutWhenUnconnected=off
  wires:
  Demux/1 -> Ir/1
  FromWs/1 -> Demux/1
  Demux/2 -> Temp/1
